simulink model "model_new_2"  (R2021a)
settings: Solver=ode23t  StartTime=0.0  StopTime=1e7  AbsTol=1e-5
values from neighbouring files (symbols this model uses):
  mp_0 = oe2mp(oe_0)    [initial_sim2.m]
  oe_0 = [a_0 e_0 incl_0 omega_0 RA_0 theta_0]    [initial_sim.m]    (also in initial_sim2.m = mp2oe(mp_0))
  oe_f = [a_f e_f incl_f omega_f RA_f theta_f]    [initial_sim.m]    (also in initial_sim2.m = mp2oe(mp_f))
  params = 0    [Combo_OT.m]
libraries: dspstat3 x6
settings Model: Creator=Mehdi  LastModifiedBy=Mehdi

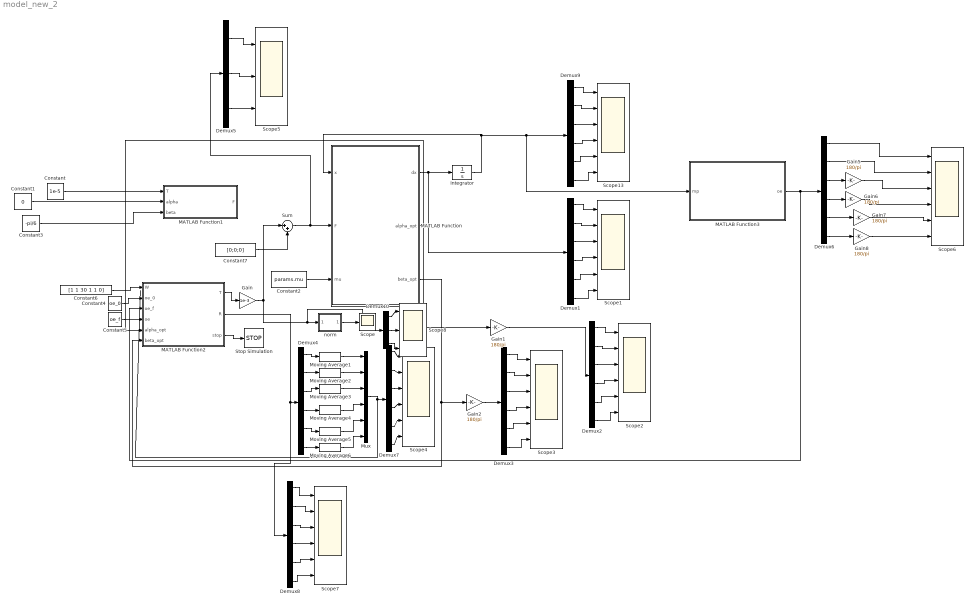
== system model_new_2 ==
  Constant : Constant  Value=1e-5
  Constant1 : Constant  Value=0
  Constant2 : Constant  Value=params.mu
  Constant3 : Constant  Value=-pi/6
  Constant4 : Constant  Value=oe_0
  Constant5 : Constant  Value=oe_f
  Constant6 : Constant  Value=[1 1 30 1 1 0]
  Constant7 : Constant  Value=[0;0;0]
  Demux{1..4,6..9} (8 alike) : Demux  Outputs=6
  Demux10 : Demux  Outputs=3
  Demux5 : Demux  Outputs=3
  Gain : Gain  Gain=1e-3
  Gain{1..2,5..8} (6 alike) : Gain  Gain=180/pi
  Integrator : Integrator  InitialCondition=mp_0
  MATLAB Function : MATLAB Function  TreatAsAtomicUnit=on
  MATLAB Function1 : MATLAB Function  TreatAsAtomicUnit=on
  MATLAB Function2 : MATLAB Function  TreatAsAtomicUnit=on
  MATLAB Function3 : MATLAB Function  TreatAsAtomicUnit=on
  Moving Average1 : dspstat3/Moving Average  Method=Sliding window  ForgettingFactorPort=off  SpecifyWindowLength=on  WindowLength=4  ForgettingFactor=0.9  SimulateUsing=Code generation
  Moving Average{2..6} (5 alike) : dspstat3/Moving Average  Method=Sliding window  ForgettingFactorPort=off  SpecifyWindowLength=on  WindowLength=20  ForgettingFactor=0.9  SimulateUsing=Code generation
  Mux : Mux  Inputs=6
  Scope : Scope
  Scope{1..4,6..7,13} (7 alike) : Scope  NumInputPorts=6
  Scope5 : Scope  NumInputPorts=3
  Scope8 : Scope  NumInputPorts=3
  Stop Simulation : Stop
  Sum : Sum  Inputs=|++
  norm : Subsystem
  wires:
  Integrator/1 -> MATLAB Function/1(x), MATLAB Function3/1(mp), Demux9/1
  Constant2/1 -> MATLAB Function/3(mu)
  Demux9/5 -> Scope13/5
  Demux9/1 -> Scope13/1
  Demux9/4 -> Scope13/4
  Demux9/3 -> Scope13/3
  Demux9/2 -> Scope13/2
  Demux9/6 -> Scope13/6
  Demux1/6 -> Scope1/6
  Demux1/2 -> Scope1/2
  Demux1/3 -> Scope1/3
  Demux1/4 -> Scope1/4
  Demux1/1 -> Scope1/1
  Demux1/5 -> Scope1/5
  Constant/1 -> MATLAB Function1/1(T)
  Constant1/1 -> MATLAB Function1/2(alpha)
  Constant3/1 -> MATLAB Function1/3(beta)
  Demux2/6 -> Scope2/6
  Demux2/2 -> Scope2/2
  Demux2/3 -> Scope2/3
  Demux2/4 -> Scope2/4
  Demux2/1 -> Scope2/1
  Demux2/5 -> Scope2/5
  MATLAB Function/2(alpha_opt) -> Gain1/1, MATLAB Function2/5(alpha_opt)
  MATLAB Function/3(beta_opt) -> MATLAB Function2/6(beta_opt), Gain2/1
  Demux3/5 -> Scope3/5
  Demux3/1 -> Scope3/1
  Demux3/4 -> Scope3/4
  Demux3/3 -> Scope3/3
  Demux3/2 -> Scope3/2
  Demux3/6 -> Scope3/6
  Constant4/1 -> MATLAB Function2/2(oe_0)
  Constant5/1 -> MATLAB Function2/3(oe_f)
  Constant6/1 -> MATLAB Function2/1(W)
  Demux5/3 -> Scope5/3
  Demux5/2 -> Scope5/2
  Demux5/1 -> Scope5/1
  MATLAB Function2/1(T) -> Gain/1
  Sum/1 -> Demux5/1, MATLAB Function/2(F)
  Constant7/1 -> Sum/2
  Gain/1 -> Sum/1, Demux10/1, norm/1(In1)
  MATLAB Function2/3(stop) -> Stop Simulation/1
  Demux6/6 -> Gain8/1
  Demux6/3 -> Gain5/1
  Demux6/4 -> Gain6/1
  Demux6/5 -> Gain7/1
  MATLAB Function3/1(oe) -> MATLAB Function2/4(oe), Demux6/1
  Demux4/1 -> Moving Average1/1
  Moving Average1/1 -> Mux/1
  Demux4/2 -> Moving Average2/1
  Demux4/3 -> Moving Average3/1
  Demux4/4 -> Moving Average4/1
  Demux4/5 -> Moving Average5/1
  Demux4/6 -> Moving Average6/1
  Moving Average2/1 -> Mux/2
  Moving Average3/1 -> Mux/3
  Moving Average4/1 -> Mux/4
  Moving Average5/1 -> Mux/5
  Moving Average6/1 -> Mux/6
  Demux7/3 -> Scope4/3
  Demux7/2 -> Scope4/2
  Demux7/4 -> Scope4/4
  Demux7/1 -> Scope4/1
  Demux7/5 -> Scope4/5
  Demux7/6 -> Scope4/6
  Mux/1 -> Demux7/1
  Demux8/4 -> Scope7/4
  Demux8/3 -> Scope7/3
  Demux8/5 -> Scope7/5
  Demux8/2 -> Scope7/2
  Demux8/6 -> Scope7/6
  Demux8/1 -> Scope7/1
  MATLAB Function2/2(R) -> Demux8/1, Demux4/1
  Gain1/1 -> Demux2/1
  MATLAB Function/1(dx) -> Demux1/1, Integrator/1
  Gain2/1 -> Demux3/1
  Demux6/1 -> Scope6/1
  Demux6/2 -> Scope6/2
  Gain5/1 -> Scope6/3
  Gain6/1 -> Scope6/4
  Gain7/1 -> Scope6/5
  Gain8/1 -> Scope6/6
  norm/1(Out1) -> Scope/1
  Demux10/2 -> Scope8/2
  Demux10/1 -> Scope8/1
  Demux10/3 -> Scope8/3

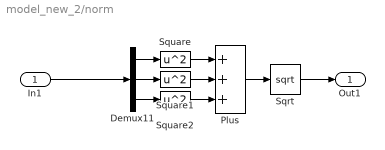
== system model_new_2/norm ==
  In1 : Inport
  Demux11 : Demux  Outputs=3
  Plus : Sum  Inputs=+++
  Sqrt : Sqrt  SaturateOnIntegerOverflow=on
  Square : Math  Operator=square  SaturateOnIntegerOverflow=on
  Square1 : Math  Operator=square  SaturateOnIntegerOverflow=on
  Square2 : Math  Operator=square  SaturateOnIntegerOverflow=on
  Out1 : Outport
  wires:
  Demux11/3 -> Square2/1
  Demux11/2 -> Square1/1
  Demux11/1 -> Square/1
  Square1/1 -> Plus/2
  Square/1 -> Plus/1
  Plus/1 -> Sqrt/1
  Sqrt/1 -> Out1/1
  Square2/1 -> Plus/3
  In1/1 -> Demux11/1

== matlab function model_new_2/MATLAB Function1 ==
  data: T input; alpha input; F output; beta input
function F = steer(T,alpha,beta)



F=T*[sin(alpha)*cos(beta);cos(alpha)*cos(beta);sin(beta)];



end

== matlab function model_new_2/MATLAB Function ==
  data: x input; F input; dx output; mu input; alpha_opt output; beta_opt output
function [dx,alpha_opt,beta_opt] = path_dynamics(x,F,mu)

% a
% ep1=e*sin(omega+OMEGA);
% ep2=e*cos(omega+OMEGA);
% zig1=tan(inc/2)*sin(OMEGA);
% zig2=tan(inc/2)*cos(OMEGA);
% lambda=theta+omega+OMEGA;


a=x(1);
ep1=x(2);
ep2=x(3);
zig1=x(4);
zig2=x(5);
lambda=x(6);

slam=sin(lambda);
clam=cos(lambda);
L=a*(1-ep1^2-ep2^2);
h=sqrt(mu*L);
r=L/(1+ep1*slam+ep2*clam);

%%% to be optimized!

a_dot=2*a^2/h*dot([ep2*slam-ep1*clam L/r 0],F);
ep1_dot=r/h*dot([-L/r*clam ep1+(1+L/r)*slam -ep2*(zig1*clam-zig2*slam)],F);
ep2_dot=r/h*dot([L/r*slam ep2+(1+L/r)*clam ep1*(zig1*clam-zig2*slam)],F);
zig1_dot=r/(2*h)*dot([0 0 (1+zig1^2+zig2^2)*slam],F);
zig2_dot=r/(2*h)*dot([0 0 (1+zig1^2+zig2^2)*clam],F);
lambda_dot=h/r^2+r/h*dot([0 0 zig2*slam-zig1*clam],F);

% dx=zeros(6,1);

dx=[a_dot;ep1_dot;ep2_dot;zig1_dot;zig2_dot;lambda_dot];



alpha_opt=zeros(6,1);
beta_opt=zeros(6,1);

alpha_opt(1)=atan(r/L*(ep2*slam-ep1*clam));
alpha_opt(2)=atan(-L*clam/(r*ep1+(r+L)*slam));
% alpha_opt(3)=atan(L*slam/(r*ep2+(r+L)*clam));


beta_opt(2)=atan(r*ep2*(zig1*clam-zig2*slam)/(L*clam*sin(alpha_opt(2))-(r*ep1+(r+L)*slam)*cos(alpha_opt(2))));
beta_opt(3)=atan(r*ep1*(zig1*clam-zig2*slam)/(L*slam*sin(alpha_opt(3))-(r*ep2+(r+L)*clam)*cos(alpha_opt(3))));

beta_opt(4)=sign(slam)*pi/2;
beta_opt(5)=sign(clam)*pi/2;

beta_opt(6)=sign(zig2*slam-zig1*clam)*pi/2;


% e=sqrt(ep1^2+ep2^2);
% inc=2*atan(sqrt(zig1^2+zig2^2));
% OMEGA=atan(zig1/zig2);
% omega=atan(ep1/ep2)-OMEGA;
% theta=lambda-atan(ep1/ep2);








end

== matlab function model_new_2/MATLAB Function2 ==
  data: W input; oe_0 input; oe_f input; oe input; alpha_opt input; beta_opt input; T output; R output; stop output
function [T,R,stop]  = Guider(W,oe_0,oe_f,oe,alpha_opt,beta_opt)


stop=0;

R=zeros(6,1);
ss=ones(6,1);

T=[0;0;0];

for i=1:6
    
    if abs(oe_f(i)-oe_0(i))>1e-5 && abs(oe_f(i)-oe(i))>1e-5
        
        R(i)=abs((oe(i)-oe_f(i))/(oe_f(i)-oe_0(i)));
        
        if R(i)>5
            R(i)=5;
        end
        
    end
end

if norm(R)<1e-3
    stop=1;
end





ss(1)=sign(oe_f(1)-oe(1));  %% sign ok
ss(2)=-sign(oe_f(2)-oe(2));  %% sign ok
ss(3)=-sign(oe_f(3)-oe(3));
ss(4)=sign(oe_f(4)-oe(4));
ss(5)=sign(oe_f(5)-oe(5));
ss(6)=sign(oe_f(6)-oe(6));

% ss=R_dot;

% ang1=rem(x(6)+2*pi,2*pi);
% if ang1>pi
%     ss(2)=-ss(2);
% alpha_opt(2)=2*pi-alpha_opt(2);
% end


for i=1:6
    %     ss=1;
    %     ang1=rem(x(6)+2*pi,2*pi);
    %     if ang1<pi
    %         alpha_opt(i)=-alpha_opt(i);
    % ss=-1;
    %     end
    
    %         ss=sign(x(i)-mp_f(i));
    %     ss=1;
    %
    % ss=-1;
    T=T+ss(i)*W(i)*R(i)*([sin(alpha_opt(i))*cos(beta_opt(i));cos(alpha_opt(i))*cos(beta_opt(i));sin(beta_opt(i))]);
    %
end

if norm(T)>0
    
    T=T./norm(T);
    
else
    T=[0;0;0];
end

end

== matlab function model_new_2/MATLAB Function3 ==
  data: mp input; oe output
function oe=mp2oe(mp)


a=mp(1);
ep1=mp(2);
ep2=mp(3);
zig1=mp(4);
zig2=mp(5);
lambda=mp(6);


% % ep1=e*sin(omega+OMEGA);
% % ep2=e*cos(omega+OMEGA);
% % zig1=tan(inc/2)*sin(OMEGA);
% % zig2=tan(inc/2)*cos(OMEGA);
% % lambda=theta+omega+OMEGA;
% %
% % mp=[a;ep1;ep2;zig1;zig2;lambda];

%%% to be optimized
e=sqrt(ep1^2+ep2^2);
inc=2*atan(sqrt(zig1^2+zig2^2));

if inc==0
    OMEGA=0;
else
    tan1=tan(inc/2);
    OMEGA=atan3(zig1/tan1,zig2/tan1);
end


% if sign(zig2)*sign(cos(OMEGA))<0 || sign(zig1)*sign(sin(OMEGA))<0
%     inc=-inc;
% end


if OMEGA>pi
    OMEGA=OMEGA-2*pi;
end

% inc=inc*(sign(zig2)*sign(cos(OMEGA)));

if e==0
    omega=0;
else
    omega=atan3(ep1/e,ep2/e)-OMEGA;
end


theta=lambda-omega-OMEGA;
if theta<0
    theta=theta+2*pi;
end

if theta>2*pi
    theta=rem(theta,2*pi);
end

oe=[a;e;inc;omega;OMEGA;theta];


end
